simulink model "chap5_3sim"  (Simulink 7.7)
settings: Solver=ode45  StartTime=0.0  StopTime=10  RelTol=1e-5
settings Model: Creator=hp  LastModifiedBy=ljk  ExtModeTrigMode=oneshot  ExtModeArmWhenConnect=off
settings DataIOCC: LimitDataPoints=off  SignalLoggingName=sigsOut
settings OptimizationCC: BooleanDataType=off  InitFltsAndDblsToZero=on
settings DebuggingCC: SaveWithParameterizedLinksMsg=none  SignalResolutionControl=TryResolveAllWithWarning  SolverPrmCheckMsg=none  MultiTaskDSMMsg=warning  MultiTaskCondExecSysMsg=none  StrictBusMsg=None
settings HardwareCC: TargetUnknown=on
settings RTWCC: IncludeERTFirstTime=on
settings GRTTargetCC: TargetFcnLib=ansi_tfl_tmw.mat

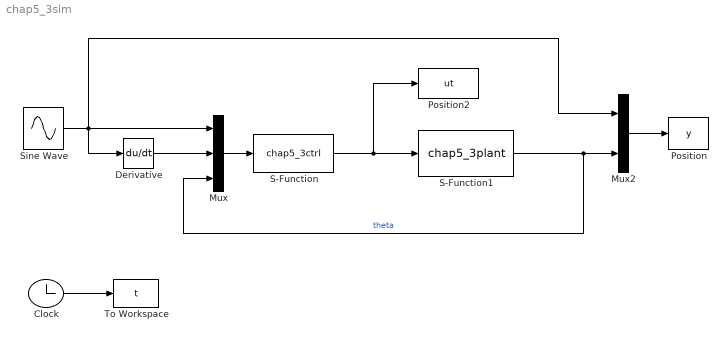
== system chap5_3sim ==
  Clock : Clock
      settings: Decimation=10
  Derivative : Derivative
  Mux : Mux  Inputs=3
  Mux2 : Mux  Inputs=2
  Position : ToWorkspace  VariableName=y  SampleTime=-1  SaveFormat=Array
  Position2 : ToWorkspace  VariableName=ut  SampleTime=-1  SaveFormat=Array
  S-Function : S-Function  FunctionName=chap5_3ctrl  EnableBusSupport=off
  S-Function1 : S-Function  FunctionName=chap5_3plant  EnableBusSupport=off
  Sine Wave : Sin  Amplitude=0.1  SampleTime=0
  To Workspace : ToWorkspace  VariableName=t  SampleTime=-1  SaveFormat=Array
  wires:
  Mux2/1 -> Position/1
  S-Function1/1 -> Mux2/2, Mux/3  "theta"
  Mux/1 -> S-Function/1
  S-Function/1 -> S-Function1/1, Position2/1
  Clock/1 -> To Workspace/1
  Sine Wave/1 -> Mux2/1, Mux/1, Derivative/1
  Derivative/1 -> Mux/2
